simulink model "FFTest"  (R2017a)
settings: Solver=ode113  StartTime=0.0  StopTime=10.0  RelTol=1e-6
values from neighbouring files (symbols this model uses):
  param = evalin('base','param')    [getSaveInfo.m]    (also in loadBackUp.m)
settings Model: Creator=www  LastModifiedBy=www
settings SolverCC: MaxConsecutiveMinStep=1000  AlgebraicLoopSolver=LineSearch
settings DataIOCC: SaveOutput=off  SignalLogging=off  DSMLogging=off  SaveTime=off

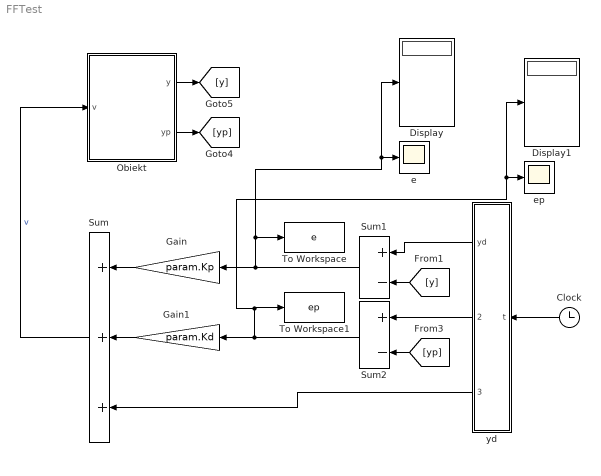
== system FFTest ==
  Clock : Clock
  Display : Display
  Display1 : Display
  Gain : Gain  Gain=param.Kp
  Gain1 : Gain  Gain=param.Kd
  Obiekt : Subsystem
  Sum : Sum  Inputs=+++
  Sum1 : Sum  Inputs=+-
  Sum2 : Sum  Inputs=+-
  To Workspace : ToWorkspace  VariableName=e  SaveFormat=Timeseries  SampleTime=-1
  To Workspace1 : ToWorkspace  VariableName=ep  SaveFormat=Timeseries  SampleTime=-1
  e : Scope
  ep : Scope
  yd : MATLAB Function  TreatAsAtomicUnit=on
  wires:
  Gain/1 -> Sum/1
  Obiekt/2(yp) -> [yp]
  Obiekt/1(y) -> [y]
  yd/2(ydp) -> Sum2/1
  [yp] -> Sum2/2
  [y] -> Sum1/2
  yd/1(yd) -> Sum1/1
  yd/3(ydpp) -> Sum/3
  Sum/1 -> Obiekt/1(v)  "v"
  Clock/1 -> yd/1(t)
  Sum1/1 -> Display/1, e/1, To Workspace/1, Gain/1
  Sum2/1 -> Display1/1, ep/1, To Workspace1/1, Gain1/1
  Gain1/1 -> Sum/2

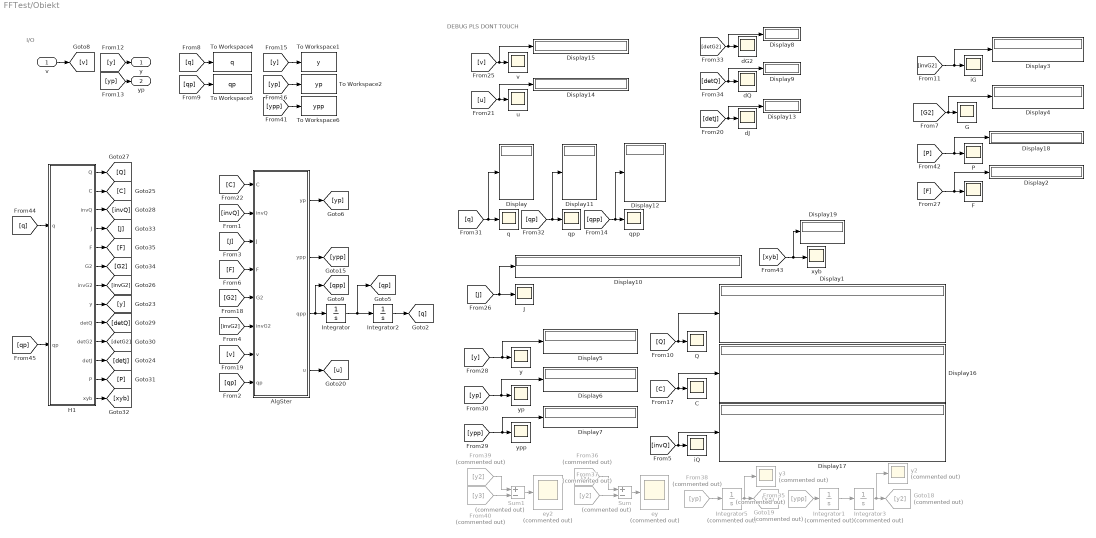
== system FFTest/Obiekt ==
  note: I/O
  note: DEBUG PLS DONT TOUCH
  v : Inport
  AlgSter : MATLAB Function  TreatAsAtomicUnit=on
  C : Scope
  Display{,1..19} (20 alike) : Display
  F : Scope
  From35 : From  Commented=on  GotoTag=ypp
  From36 : From  Commented=on  GotoTag=y
  From37 : From  Commented=on  GotoTag=y2
  From38 : From  Commented=on  GotoTag=yp
  From39 : From  Commented=on  GotoTag=y2
  From40 : From  Commented=on  GotoTag=y3
  G : Scope
  Goto18 : Goto  Commented=on  GotoTag=y2
  Goto19 : Goto  Commented=on  GotoTag=y3
  H1 : MATLAB Function  TreatAsAtomicUnit=on
  Integrator : Integrator  InitialCondition=param.initCond.qp0
  Integrator1 : Integrator  Commented=on  InitialCondition=param.initCond.Yp0
  Integrator2 : Integrator  InitialCondition=param.initCond.q0
  Integrator3 : Integrator  Commented=on  InitialCondition=param.initCond.Y0
  Integrator5 : Integrator  Commented=on  InitialCondition=param.initCond.Y0
  J : Scope
  P : Scope
  Q : Scope
  Sum : Sum  Commented=on  Inputs=+-
  Sum1 : Sum  Commented=on  Inputs=+-
  To Workspace1 : ToWorkspace  VariableName=y  SaveFormat=Timeseries  SampleTime=-1
  To Workspace2 : ToWorkspace  VariableName=yp  SaveFormat=Timeseries  SampleTime=-1
  To Workspace4 : ToWorkspace  VariableName=q  SaveFormat=Timeseries  SampleTime=-1
  To Workspace5 : ToWorkspace  VariableName=qp  SaveFormat=Timeseries  SampleTime=-1
  To Workspace6 : ToWorkspace  VariableName=ypp  SaveFormat=Timeseries  SampleTime=-1
  dG2 : Scope
  dJ : Scope
  dQ : Scope
  ey : Scope  Commented=on
  ey2 : Scope  Commented=on
  iG : Scope
  iQ : Scope
  q : Scope
  qp : Scope
  qpp : Scope
  "u  " : Scope
  "v  " : Scope
  xyb : Scope
  "y " : Scope
  y2 : Scope  Commented=on
  y3 : Scope  Commented=on
  "yp " : Scope
  ypp : Scope
  y : Outport
  yp : Outport  Port=2
  wires:
  v/1 -> [v]
  [G2] -> AlgSter/5(G2)
  [J] -> AlgSter/3(J)
  [v] -> AlgSter/7(v)
  [q] -> To Workspace4/1
  [yp] -> yp/1
  [yp] -> To Workspace2/1
  [y] -> To Workspace1/1
  AlgSter/2(ypp) -> [ypp]
  [y] -> y/1
  [qp] -> To Workspace5/1
  AlgSter/1(yp) -> [yp]
  [F] -> AlgSter/4(F)
  [C] -> AlgSter/1(C)
  [invQ] -> AlgSter/2(invQ)
  [qp] -> AlgSter/8(qp)
  [Q] -> Display1/1, Q/1
  [C] -> Display16/1, C/1
  [invQ] -> Display17/1, iQ/1
  [J] -> Display10/1, J/1
  [y] -> Display5/1, "y "/1
  [yp] -> Display6/1, "yp "/1
  [ypp] -> Display7/1, ypp/1
  [q] -> Display/1, q/1
  [qp] -> qp/1, Display11/1
  [detG2] -> Display8/1, dG2/1
  [detQ] -> Display9/1, dQ/1
  Integrator1/1 -> Integrator3/1
  From35/1 -> Integrator1/1
  Integrator3/1 -> y2/1, Goto18/1
  From36/1 -> Sum/1
  From37/1 -> Sum/2
  Sum/1 -> ey/1
  From38/1 -> Integrator5/1
  Integrator5/1 -> y3/1, Goto19/1
  From40/1 -> Sum1/2
  From39/1 -> Sum1/1
  Sum1/1 -> ey2/1
  [ypp] -> To Workspace6/1
  [F] -> Display2/1, F/1
  AlgSter/3(qpp) -> [qpp], Integrator/1
  Integrator/1 -> [qp], Integrator2/1
  Integrator2/1 -> [q]
  [invG2] -> AlgSter/6(invG2)
  [invG2] -> Display3/1, iG/1
  [G2] -> Display4/1, G/1
  [qpp] -> Display12/1, qpp/1
  [detJ] -> Display13/1, dJ/1
  [u] -> Display14/1, "u  "/1
  [v] -> Display15/1, "v  "/1
  AlgSter/4(u) -> [u]
  [P] -> Display18/1, P/1
  [xyb] -> Display19/1, xyb/1
  H1/13(xyb) -> [xyb]
  H1/12(P) -> [P]
  H1/11(detJ) -> [detJ]
  H1/10(detG2) -> [detG2]
  H1/3(invQ) -> [invQ]
  H1/4(J) -> [J]
  [q] -> H1/1(q)
  H1/1(Q) -> [Q]
  H1/9(detQ) -> [detQ]
  H1/8(y) -> [y]
  H1/7(invG2) -> [invG2]
  H1/5(F) -> [F]
  H1/2(C) -> [C]
  [qp] -> H1/2(qp)
  H1/6(G2) -> [G2]

== matlab function FFTest/Obiekt/H1 ==
  data: Q output; C output; q input; qp input; invQ output; J output; F output; G2 output; invG2 output; y output; detQ output; detG2 output; detJ output; P output; xyb output
function [Q,C,invQ,J,F,G2,invG2,y,detQ,detG2,detJ,P,xyb] = fcn(q,qp)

c0=cos(q(3));
c1=cos(q(4));
c2=cos(q(5));
s0=sin(q(3));
s1=sin(q(4));
s2=sin(q(5));
s12=sin(q(4)+q(5));
c12=cos(q(4)+q(5));
xyb=[1;1];

y=[q(1)+(5/8).*cos(q(4)+q(3))+(7/8).*cos(q(4)+q(5)+q(3)),q(2)+(5/8).*sin(q(4)+q(3))+( ...
  7/8).*sin(q(4)+q(5)+q(3))];
J=[1,0,(1/8).*((-5).*sin(q(4)+q(3))+(-7).*sin(q(4)+q(5)+q(3))),(1/8).*((-5).* ...
  sin(q(4)+q(3))+(-7).*sin(q(4)+q(5)+q(3))),(-7/8).*sin(q(4)+q(5)+q(3));0,1,(1/8).*(5.* ...
  cos(q(4)+q(3))+7.*cos(q(4)+q(5)+q(3))),(1/8).*(5.*cos(q(4)+q(3))+7.*cos(q(4)+q(5)+q(3))),( ...
  7/8).*cos(q(4)+q(5)+q(3))];
F=[((-737)+225.*cos(2.*q(5))).^(-1).*((-25).*(qp(3)+qp(4)).^2.*cos(q(4)+q(3))+( ...
  -75).*(qp(3)+qp(4)+qp(5)).^2.*cos(q(4)+(-1).*q(5)+q(3))+523.*qp(3).^2.*cos(q(4)+q(5)+ ...
  q(3))+1046.*qp(3).*qp(4).*cos(q(4)+q(5)+q(3))+523.*qp(4).^2.*cos(q(4)+q(5)+q(3))+1046.* ...
  qp(3).*qp(5).*cos(q(4)+q(5)+q(3))+1046.*qp(4).*qp(5).*cos(q(4)+q(5)+q(3))+523.*qp(5).^2.* ...
  cos(q(4)+q(5)+q(3))+345.*qp(3).^2.*cos(q(4)+2.*q(5)+q(3))+690.*qp(3).*qp(4).*cos(q(4)+ ...
  2.*q(5)+q(3))+345.*qp(4).^2.*cos(q(4)+2.*q(5)+q(3)));((-737)+225.*cos(2.*q(5))).^( ...
  -1).*((-25).*(qp(3)+qp(4)).^2.*sin(q(4)+q(3))+(-75).*(qp(3)+qp(4)+qp(5)).^2.*sin( ...
  q(4)+(-1).*q(5)+q(3))+523.*qp(3).^2.*sin(q(4)+q(5)+q(3))+1046.*qp(3).*qp(4).*sin(q(4)+ ...
  q(5)+q(3))+523.*qp(4).^2.*sin(q(4)+q(5)+q(3))+1046.*qp(3).*qp(5).*sin(q(4)+q(5)+q(3))+ ...
  1046.*qp(4).*qp(5).*sin(q(4)+q(5)+q(3))+523.*qp(5).^2.*sin(q(4)+q(5)+q(3))+345.* ...
  qp(3).^2.*sin(q(4)+2.*q(5)+q(3))+690.*qp(3).*qp(4).*sin(q(4)+2.*q(5)+q(3))+345.* ...
  qp(4).^2.*sin(q(4)+2.*q(5)+q(3)))];
G2=[((-481)+225.*c2.^2).^(-1).*(39.*sin(q(4)+q(3))+(-63).*c2.*sin(q(4)+q(5)+ ...
  q(3))),(3/5).*((-481)+225.*c2.^2).^(-1).*((-5).*(13+15.*c2).*sin( ...
  q(4)+q(3))+7.*(37+15.*c2).*sin(q(4)+q(5)+q(3)));3.*((-737)+225.*cos(2.*q(5))) ...
  .^(-1).*((-5).*cos(q(4)+q(3))+21.*cos(q(4)+2.*q(5)+q(3))),(3/5).*((-481)+225.* ...
  c2.^2).^(-1).*((65+75.*c2).*cos(q(4)+q(3))+(-7).*(37+15.*c2).*cos( ...
  q(4)+q(5)+q(3)))];
G2dot=[(481+(-225).*c2.^2).^(-2).*(450.*c2.*qp(5).*s2.*(39.*sin(q(4)+q(3))+( ...
  -63).*c2.*sin(q(4)+q(5)+q(3)))+((-481)+225.*c2.^2).*(39.*(qp(3)+qp(4)).* ...
  cos(q(4)+q(3))+(-63).*c2.*(qp(3)+qp(4)+qp(5)).*cos(q(4)+q(5)+q(3))+63.*qp(5).*s2.* ...
  sin(q(4)+q(5)+q(3)))),(1/5).*(481+(-225).*c2.^2).^(-2).*(450.*c2.*qp(5).* ...
  s2.*((-15).*(13+15.*c2).*sin(q(4)+q(3))+21.*(37+15.*c2).*sin(q(4)+q(5)+ ...
  q(3)))+3.*((-481)+225.*c2.^2).*((-5).*(13+15.*c2).*(qp(3)+qp(4)).*cos( ...
  q(4)+q(3))+7.*(37+15.*c2).*(qp(3)+qp(4)+qp(5)).*cos(q(4)+q(5)+q(3))+75.*qp(5).*s2.* ...
  sin(q(4)+q(3))+(-105).*qp(5).*s2.*sin(q(4)+q(5)+q(3))));3.*(737+(-225).*cos(2.* ...
  q(5))).^(-2).*(450.*qp(5).*((-5).*cos(q(4)+q(3))+21.*cos(q(4)+2.*q(5)+q(3))).*sin( ...
  2.*q(5))+((-737)+225.*cos(2.*q(5))).*(5.*(qp(3)+qp(4)).*sin(q(4)+q(3))+(-21).*( ...
  qp(3)+qp(4)+2.*qp(5)).*sin(q(4)+2.*q(5)+q(3)))),(3/5).*(481+(-225).*c2.^2).^( ...
  -2).*(450.*c2.*qp(5).*s2.*((65+75.*c2).*cos(q(4)+q(3))+(-7).*(37+15.* ...
  c2).*cos(q(4)+q(5)+q(3)))+((-481)+225.*c2.^2).*((-75).*qp(5).*s2.*cos( ...
  q(4)+q(3))+105.*qp(5).*s2.*cos(q(4)+q(5)+q(3))+(-5).*(13+15.*c2).*(qp(3)+qp(4)).* ...
  sin(q(4)+q(3))+7.*(37+15.*c2).*(qp(3)+qp(4)+qp(5)).*sin(q(4)+q(5)+q(3))))];
 
disturb=[0 0;0 0];
if abs(det(G2))>0.0001
else
   disturb=1*[sign(G2dot(1,1)) 0;
                0 sign(G2dot(2,2))];
end
G2=G2+disturb;
    
invG2=inv(G2);
P=[(1/8).*((-5).*(qp(3)+qp(4)).^2.*cos(q(4)+q(3))+(-7).*(qp(3)+qp(4)+qp(5)).^2.* ...
  cos(q(4)+q(5)+q(3)));(1/8).*((-5).*(qp(3)+qp(4)).^2.*sin(q(4)+q(3))+(-7).*(qp(3)+ ...
  qp(4)+qp(5)).^2.*sin(q(4)+q(5)+q(3)))];
Q=[40,0,0,0,0;0,40,0,0,0;0,0,(5/12).*(49+15.*c2),(25/12).*(5+3.* ...
  c2),(5/24).*(13+15.*c2);0,0,(25/12).*(5+3.*c2),(25/12).*(5+3.* ...
  c2),(5/24).*(13+15.*c2);0,0,(5/24).*(13+15.*c2),(5/24).*(13+ ...
  15.*c2),(65/24)];
C=[0,0,0,0,0;0,0,0,0,0;0,0,(-25/8).*qp(5).*s2,(-25/8).*qp(5).*s2,( ...
  -25/8).*(qp(3)+qp(4)+qp(5)).*s2;0,0,(-25/8).*qp(5).*s2,(-25/8).*qp(5).* ...
  s2,(-25/8).*(qp(3)+qp(4)+qp(5)).*s2;0,0,(25/8).*(qp(3)+qp(4)).*s2,(25/8) ...
  .*(qp(3)+qp(4)).*s2,0];
invQ=[(1/40),0,0,0,0;0,(1/40),0,0,0;0,0,(1/10),(-1/10),0;0,0,(-1/10),( ...
  962+(-450).*c2.^2).^(-1).*(221+(-45).*c2.^2),(48/5).*(13+15.* ...
  c2).*((-737)+225.*cos(2.*q(5))).^(-1);0,0,0,(48/5).*(13+15.*c2).*( ...
  (-737)+225.*cos(2.*q(5))).^(-1),(-96).*(5+3.*c2).*((-737)+225.*cos( ...
  2.*q(5))).^(-1)];



detQ=det(Q);
detJ=1337;
detG2=det(G2);

== matlab function FFTest/Obiekt/AlgSter ==
  data: C input; invQ input; yp output; ypp output; J input; F input; G2 input; invG2 input; v input; qp input; qpp output; u output
function [yp,ypp,qpp,u] = fcn(C,invQ,J,F,G2,invG2,v,qp)

yp=J*qp;
ypp=F+G2*v;

u=invG2*(-F+v);
qpp=invQ*([0;0;0;u]-C*qp);

== matlab function FFTest/yd ==
  data: yd output; ydp output; ydpp output; t input
function [yd,ydp, ydpp] = fcn(t)
% y: 1:atan 2:poly   3:sin
%   4:cos  5:const1 6:const2 7:ln
y1=3;
y2=4;

const1=1.6;
const2=0;

dln=1;
lna=0.01;
lnb=30;
lndt=1;

a=1;
b=1;

p4=0;
p3=0;
p2=0;
p1=0.5;
p0=0;

sina=1;
sinb=1;

cosa=1;
cosb=1;

ln=dln+lna*log(lnb*(t+lndt));
arctg=a*atan(b*t);
poly=p4*t^4+p3*t^3+p2*t^2+p1*t+p0;
sinn=sina*sin(sinb*t);
coss=cosa*cos(cosb*t);

lnp=lna/(t+lndt);
lnpp=-lna/(t+lndt)^2;

polyp=4*p4*t^3+3*p3*t^2+2*p2*t+p1;
polypp=12*p4*t^2+6*p3*t+2*p2;

arctgp=(a*b)/(b^2*t^2+1);
arctgpp=-(2*a*b^3*t)/(b^2*t^2+1)^2;

sinp=sina*sinb*cos(sinb*t);
sinpp=-sina*sinb^2*sin(sinb*t);

cosp=-cosa*cosb*sin(cosb*t);
cospp=-cosa*cosb^2*cos(cosb*t);

f=[arctg,poly,sinn,coss,const1,const2,ln];
fp=[arctgp,polyp,sinp,cosp,0,0,lnp];
fpp=[arctgpp,polypp,sinpp,cospp,0,0,lnpp];

yd=[f(y1);
    f(y2)];

ydp=[fp(y1);
   fp(y2)];

ydpp=[fpp(y1);
     fpp(y2)];
